simulink library "library_schuettgut"  (R2020a)
settings: Solver=VariableStepAuto  StartTime=0.0  StopTime=10.0  RelTol=1e-3
undefined symbols (not defined in the file or in its folder): delay, gain, OK
libraries: simulink x7, $bdroot x3
settings Model: Creator=Jonathan  LastModifiedBy=Jonathan

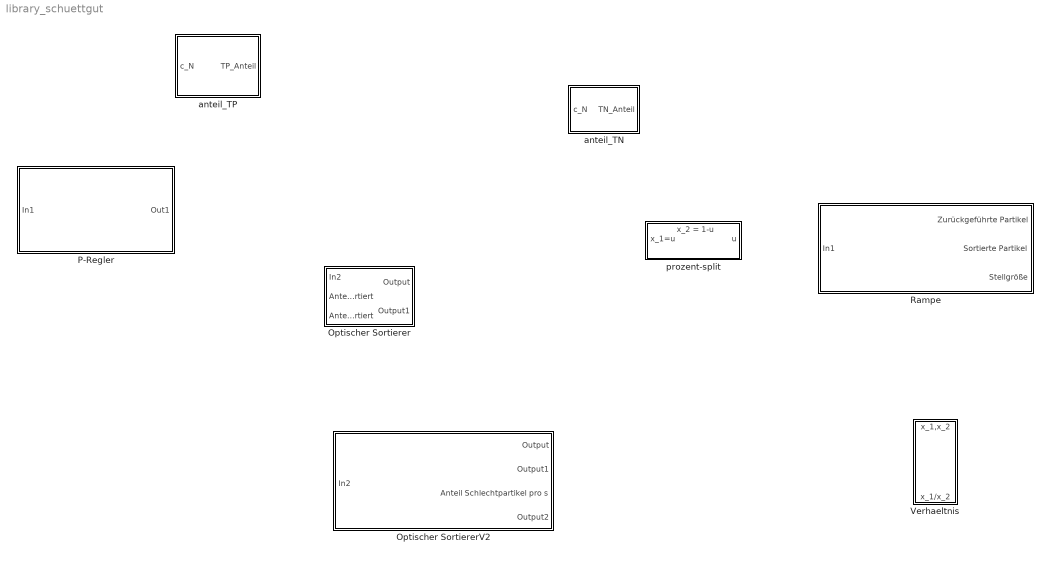
== system library_schuettgut ==
  Optischer Sortierer : Subsystem
  Optischer SortiererV2 : Subsystem  AncestorBlock=library_schuettgut/Optischer Sortierer
  P-Regler : Subsystem  mask{gain=1, delay=1, TrueorFalse=0}
      mask prompts: delay "Time Delay"; TrueorFalse "Reglerinput"
  Rampe : Subsystem  Tag=Rampe  mask{OK=OK, gain=gain, delay=delay, TrueorFalse=0, errorP=0, errorN=0}
      mask prompts: OK "Abstand OS Kamera"; gain "Regler-Gain:"; delay "Regler-Totzeit"; TrueorFalse "Reglerinput:"; errorP "Reglerfehler Gutpartikel:"; errorN "Reglerfehler Schlechtpartikel"
      mask help:
      | Reglerinput:
      | Reglerinput = 1 => Gutpartikel pro s wird als Reglerinput verwendet
      | Reglerinput = 0 => Schlechtpartike pro s wird als Reglerinput verwendet
      mask TypeOptions TrueorFalse: 0 | 1
  "Verhaeltnis " : Subsystem
  anteil_TN : MATLAB Function  TreatAsAtomicUnit=on
  anteil_TP : MATLAB Function  TreatAsAtomicUnit=on
  prozent-split : Subsystem
      settings: PortSchema="{\"entries\":[{\"content\":{\"sides\":[{\"content\":{\"connectorIds\":[\"In1\"]},\"type\":\"ConnectorPlacement.EquallySpacedRectSide\",\"uuid\":\"ab8511c8-9f1d-48ad-bf24-85fd477f0bdd\"},{\"content\":{\"connectorIds\":[\"Out1\"],\"side\":\"RIGHT\"},\"type\":\"ConnectorPlacement.EquallySpacedRectSide\",\"uuid\":\"9ac1a19a-8176-444e-9f4d-7beffa0184e3\"},{\"content\":{\"connectorIds\":[\"Out2\"],\"side\":\"TOP\"},\"type\":\"ConnectorPlacement.EquallySpacedRectSide\",\"uuid\":\"376c2400-f821-4649-ab16-706a2da6117b\"}]},\"type\":\"ConnectorPlacement.EquallySpacedConnector\",\"uuid\":\"f6e72b2d-0467-4732-a018-d51f3a5db703\"}],\"packageUris\":[\"http://schema.mathworks.com/mf0/Connector/19700101\"],\"version\":\"1.0\"}"

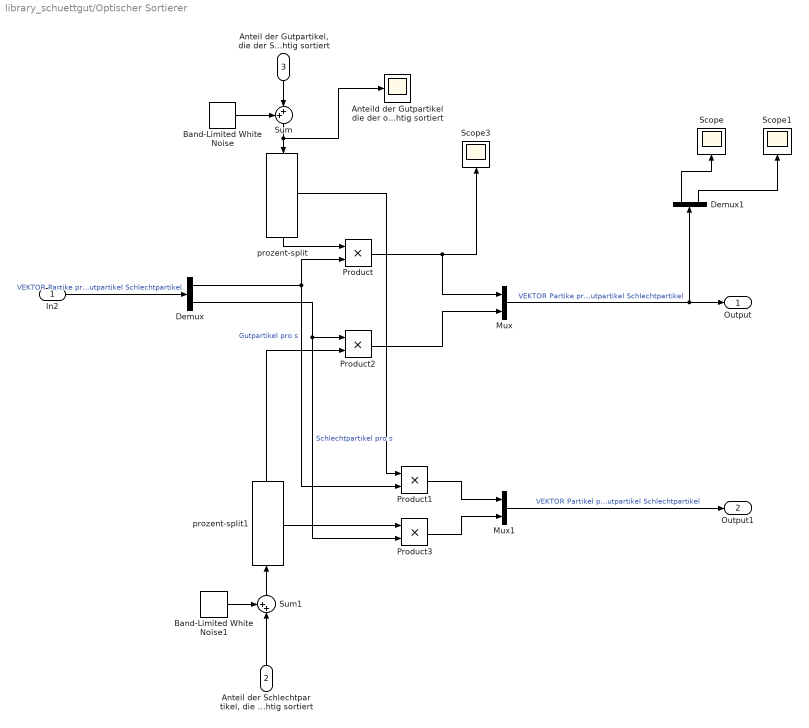
== system library_schuettgut/Optischer Sortierer ==
  In2 : Inport
  "Anteil der Schlechtpartikel, die der Sortierer richtig sortiert " : Inport  Port=2
  "Anteil der Gutpartikel, die der Sortierer richtig sortiert" : Inport  Port=3
  Anteild der Gutpartikel die der optische Sortiererrichtig richtig sortiert : Scope
  Band-Limited White Noise : simulink/Sources/Band-Limited White Noise  Cov=[0.0001]  Ts=0.1  seed=[23341]
  Band-Limited White Noise1 : simulink/Sources/Band-Limited White Noise  Cov=[0.0001]  Ts=0.1  seed=[23341]
  Demux : Demux  Outputs=2
  Demux1 : Demux  Outputs=2
  Mux : Mux  Inputs=2
  Mux1 : Mux  Inputs=2
  Product{,1..3} (4 alike) : Product
  Scope : Scope
  Scope1 : Scope
  Scope3 : Scope
  Sum : Sum  Inputs=++|
  Sum1 : Sum  Inputs=++|
  prozent-split : $bdroot/prozent-split  SystemSampleTime=-1  Latency=0  AutoFrameSizeCalculation=off
      settings: PortSchema="{\"entries\":[{\"content\":{\"sides\":[{\"content\":{\"connectorIds\":[\"In1\"]},\"type\":\"ConnectorPlacement.EquallySpacedRectSide\",\"uuid\":\"ab8511c8-9f1d-48ad-bf24-85fd477f0bdd\"},{\"content\":{\"connectorIds\":[\"Out1\"],\"side\":\"RIGHT\"},\"type\":\"ConnectorPlacement.EquallySpacedRectSide\",\"uuid\":\"9ac1a19a-8176-444e-9f4d-7beffa0184e3\"},{\"content\":{\"connectorIds\":[\"Out2\"],\"side\":\"TOP\"},\"type\":\"ConnectorPlacement.EquallySpacedRectSide\",\"uuid\":\"376c2400-f821-4649-ab16-706a2da6117b\"}]},\"type\":\"ConnectorPlacement.EquallySpacedConnector\",\"uuid\":\"f6e72b2d-0467-4732-a018-d51f3a5db703\"}],\"packageUris\":[\"http://schema.mathworks.com/mf0/Connector/19700101\"],\"version\":\"1.0\"}"
  prozent-split1 : $bdroot/prozent-split  SystemSampleTime=-1  Latency=0  AutoFrameSizeCalculation=off
      settings: PortSchema="{\"entries\":[{\"content\":{\"sides\":[{\"content\":{\"connectorIds\":[\"In1\"]},\"type\":\"ConnectorPlacement.EquallySpacedRectSide\",\"uuid\":\"ab8511c8-9f1d-48ad-bf24-85fd477f0bdd\"},{\"content\":{\"connectorIds\":[\"Out1\"],\"side\":\"RIGHT\"},\"type\":\"ConnectorPlacement.EquallySpacedRectSide\",\"uuid\":\"9ac1a19a-8176-444e-9f4d-7beffa0184e3\"},{\"content\":{\"connectorIds\":[\"Out2\"],\"side\":\"TOP\"},\"type\":\"ConnectorPlacement.EquallySpacedRectSide\",\"uuid\":\"376c2400-f821-4649-ab16-706a2da6117b\"}]},\"type\":\"ConnectorPlacement.EquallySpacedConnector\",\"uuid\":\"f6e72b2d-0467-4732-a018-d51f3a5db703\"}],\"packageUris\":[\"http://schema.mathworks.com/mf0/Connector/19700101\"],\"version\":\"1.0\"}"
  Output : Outport
  Output1 : Outport  Port=2
  wires:
  Demux1/1 -> Scope/1
  Demux1/2 -> Scope1/1
  Product3/1 -> Mux1/2
  Product1/1 -> Mux1/1
  prozent-split1/2 -> Product3/1
  prozent-split1/1 -> Product2/2
  Demux/2 -> Product2/1, Product3/2  "Schlechtpartikel pro s"
  Product2/1 -> Mux/2
  Band-Limited White Noise1/1 -> Sum1/1
  Sum1/1 -> prozent-split1/1
  "Anteil der Schlechtpartikel, die der Sortierer richtig sortiert "/1 -> Sum1/2
  Product/1 -> Mux/1, Scope3/1
  prozent-split/2 -> Product1/1
  Sum/1 -> Anteild der Gutpartikel die der optische Sortiererrichtig richtig sortiert/1, prozent-split/1
  Band-Limited White Noise/1 -> Sum/1
  prozent-split/1 -> Product/1
  Demux/1 -> Product/2, Product1/2  "Gutpartikel pro s"
  Mux/1 -> Output/1, Demux1/1  "VEKTOR Partike pro s in der Gutfraktion: Gutpartikel Schlechtpartikel"
  Mux1/1 -> Output1/1  "VEKTOR Partikel pro s in der Schlechtfraktion: Gutpartikel Schlechtpartikel"
  In2/1 -> Demux/1  "VEKTOR Partike pro s: Gutpartikel Schlechtpartikel"
  "Anteil der Gutpartikel, die der Sortierer richtig sortiert"/1 -> Sum/2

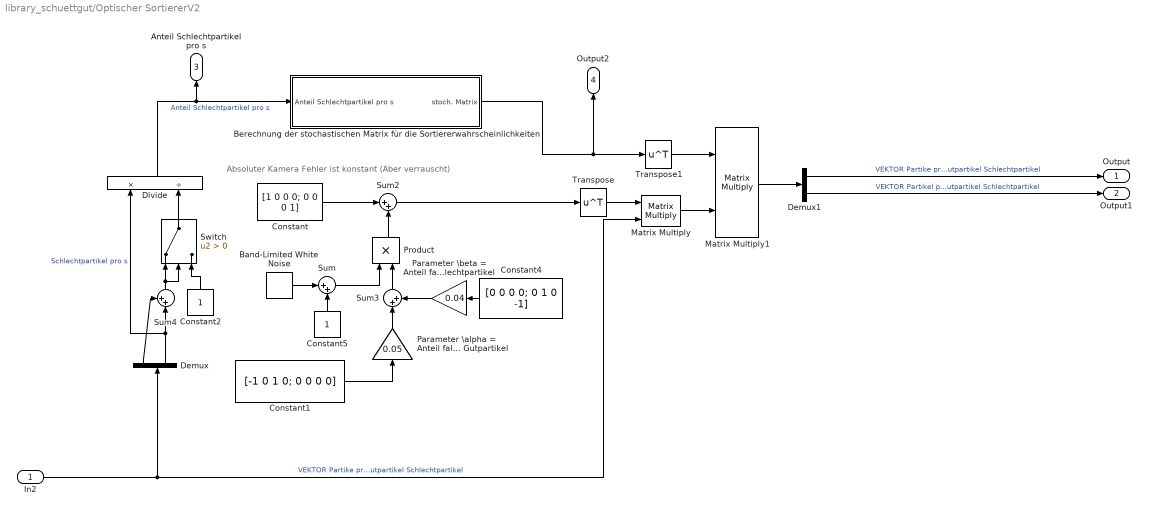
== system library_schuettgut/Optischer SortiererV2 ==
  note: Absoluter Kamera Fehler ist konstant (Aber verrauscht)
  In2 : Inport
  Band-Limited White Noise : simulink/Sources/Band-Limited White Noise  Cov=[0]  Ts=0.1  seed=[23341]
  Berechnung der stochastischen Matrix für die Sortiererwahrscheinlichkeiten : Subsystem
  Constant : Constant  Value=[1 0 0 0; 0 0 0 1]
  Constant1 : Constant  Value=[-1 0 1 0; 0 0 0 0]
  Constant2 : Constant
  Constant4 : Constant  Value=[0 0 0 0; 0 1 0 -1]
  Constant5 : Constant
  Demux : Demux  Outputs=2
  Demux1 : Demux  Outputs=2
  Divide : Product  Inputs=*/
  Matrix Multiply : Product  Multiplication=Matrix(*)
  Matrix Multiply1 : Product  Multiplication=Matrix(*)
  Parameter \alpha = Anteil falsch detektierter Gutpartikel : Gain  Gain=0.05
  Parameter \beta = Anteil falsch detektierter Schlechtpartikel : Gain  Gain=0.04
  Product : Product
  Sum : Sum  Inputs=|++
  Sum2 : Sum  Inputs=|++
  Sum3 : Sum  Inputs=|++
  Sum4 : Sum  Inputs=++|
  Switch : Switch  Criteria=u2 > Threshold
  Transpose : Math  Operator=transpose  SaturateOnIntegerOverflow=on
  Transpose1 : Math  Operator=transpose  SaturateOnIntegerOverflow=on
  Output : Outport
  Output1 : Outport  Port=2
  Anteil Schlechtpartikel pro s : Outport  Port=3
  Output2 : Outport  Port=4
  wires:
  Demux1/1 -> Output/1  "VEKTOR Partike pro s in der Gutfraktion: Gutpartikel Schlechtpartikel"
  Demux1/2 -> Output1/1  "VEKTOR Partikel pro s in der Schlechtfraktion: Gutpartikel Schlechtpartikel"
  Transpose/1 -> Matrix Multiply/1
  Matrix Multiply/1 -> Matrix Multiply1/2
  Transpose1/1 -> Matrix Multiply1/1
  Matrix Multiply1/1 -> Demux1/1
  In2/1 -> Matrix Multiply/2, Demux/1  "VEKTOR Partike pro s: Gutpartikel Schlechtpartikel"
  Constant1/1 -> Parameter \alpha = Anteil falsch detektierter Gutpartikel/1
  Sum2/1 -> Transpose/1
  Demux/2 -> Divide/1, Sum4/2  "Schlechtpartikel pro s"
  Sum4/1 -> Switch/2, Switch/1
  Demux/1 -> Sum4/1
  Divide/1 -> Anteil Schlechtpartikel pro s/1, Berechnung der stochastischen Matrix für die Sortiererwahrscheinlichkeiten/1(Anteil Schlechtpartikel pro s)  "Anteil Schlechtpartikel pro s"
  Berechnung der stochastischen Matrix für die Sortiererwahrscheinlichkeiten/1(stoch. Matrix) -> Output2/1, Transpose1/1
  Constant4/1 -> Parameter \beta = Anteil falsch detektierter Schlechtpartikel/1
  Parameter \beta = Anteil falsch detektierter Schlechtpartikel/1 -> Sum3/2
  Parameter \alpha = Anteil falsch detektierter Gutpartikel/1 -> Sum3/1
  Sum3/1 -> Product/2
  Constant/1 -> Sum2/1
  Product/1 -> Sum2/2
  Sum/1 -> Product/1
  Band-Limited White Noise/1 -> Sum/1
  Constant5/1 -> Sum/2
  Switch/1 -> Divide/2
  Constant2/1 -> Switch/3

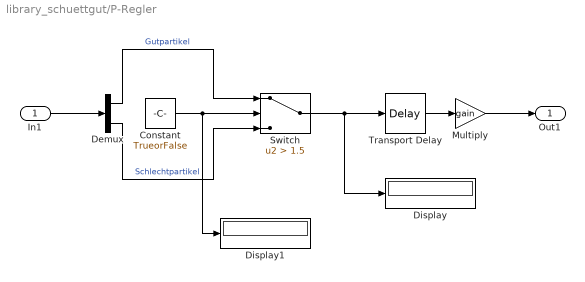
== system library_schuettgut/P-Regler ==
  In1 : Inport
  Constant : Constant  Value=TrueorFalse
  Demux : Demux  Outputs=2
  Display : Display
  Display1 : Display
  Multiply : Gain  Gain=gain
  Switch : Switch  Criteria=u2 > Threshold  Threshold=1.5
  Transport Delay : TransportDelay  DelayTime=delay
  Out1 : Outport
  wires:
  In1/1 -> Demux/1
  Demux/2 -> Switch/3  "Schlechtpartikel"
  Transport Delay/1 -> Multiply/1
  Multiply/1 -> Out1/1
  Constant/1 -> Display1/1, Switch/2
  Demux/1 -> Switch/1  "Gutpartikel"
  Switch/1 -> Display/1, Transport Delay/1

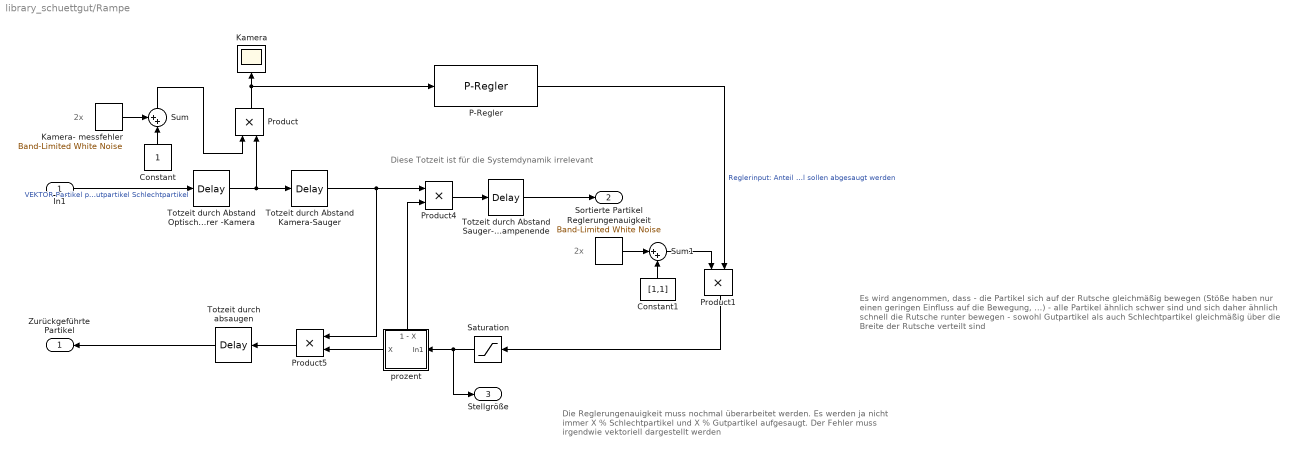
== system library_schuettgut/Rampe ==
  note: Diese Totzeit ist für die Systemdynamik irrelevant
  note: 2x
  note: 2x
  note: Die Reglerungenauigkeit muss nochmal überarbeitet werden.
      | Es werden ja nicht immer X % Schlechtpartikel und X %
      | Gutpartikel aufgesaugt. Der Fehler muss irgendwie vektoriell dargestellt werden
  note: Es wird angenommen, dass
      | - die Partikel sich auf der Rutsche gleichmäßig bewegen (Stöße haben nur einen geringen Einfluss auf die Bewegung, ...)
      | - alle Partikel ähnlich schwer sind und sich daher ähnlich schnell die Rutsche runter bewegen
      | - sowohl Gutpartikel als auch Schlechtpartikel gleichmäßig über die Breite der Rutsche verteilt sind
  In1 : Inport
  Constant : Constant
  Constant1 : Constant  Value=[1,1]
  Kamera : Scope
  Kamera- messfehler : simulink/Sources/Band-Limited White Noise  Cov=[0.0001 0.00011]  Ts=0.1  seed=[23341]
  P-Regler : $bdroot/P-Regler  gain=gain  delay=delay  TrueorFalse=TrueorFalse
  Product : Product
  Product1 : Product  OutMin=0  OutMax=1
  Product4 : Product
  Product5 : Product
  Reglerungenauigkeit : simulink/Sources/Band-Limited White Noise  Cov=[errorP errorN]  Ts=0.1  seed=[23341]
  Saturation : Saturate  UpperLimit=0.9  LowerLimit=0
  Sum : Sum  Inputs=++|
  Sum1 : Sum  Inputs=|++
  Totzeit durch Abstand Optischer Sortierer -Kamera : TransportDelay  DelayTime=OK
  Totzeit durch Abstand Kamera-Sauger : TransportDelay
  Totzeit durch Abstand Sauger-Rampenende : TransportDelay
  Totzeit durch absaugen : TransportDelay
  prozent : Subsystem
      settings: PortSchema="{\"entries\":[{\"content\":{\"sides\":[{\"content\":{\"connectorIds\":[\"In1\"]},\"type\":\"ConnectorPlacement.EquallySpacedRectSide\",\"uuid\":\"ab8511c8-9f1d-48ad-bf24-85fd477f0bdd\"},{\"content\":{\"connectorIds\":[\"Out1\"],\"side\":\"RIGHT\"},\"type\":\"ConnectorPlacement.EquallySpacedRectSide\",\"uuid\":\"9ac1a19a-8176-444e-9f4d-7beffa0184e3\"},{\"content\":{\"connectorIds\":[\"Out2\"],\"side\":\"TOP\"},\"type\":\"ConnectorPlacement.EquallySpacedRectSide\",\"uuid\":\"376c2400-f821-4649-ab16-706a2da6117b\"}]},\"type\":\"ConnectorPlacement.EquallySpacedConnector\",\"uuid\":\"f6e72b2d-0467-4732-a018-d51f3a5db703\"}],\"packageUris\":[\"http://schema.mathworks.com/mf0/Connector/19700101\"],\"version\":\"1.0\"}"
  Zurückgeführte Partikel : Outport
  Sortierte Partikel : Outport  Port=2
  Stellgröße : Outport  Port=3
  wires:
  prozent/2(1 - X) -> Product4/2
  prozent/1(X) -> Product5/2
  In1/1 -> Totzeit durch Abstand Optischer Sortierer -Kamera/1  "VEKTOR Partikel pro s: Gutpartikel Schlechtpartikel"
  Product/1 -> Kamera/1, P-Regler/1
  Totzeit durch absaugen/1 -> Zurückgeführte Partikel/1
  Totzeit durch Abstand Optischer Sortierer -Kamera/1 -> Totzeit durch Abstand Kamera-Sauger/1, Product/2
  Product5/1 -> Totzeit durch absaugen/1
  Totzeit durch Abstand Kamera-Sauger/1 -> Product4/1, Product5/1
  Totzeit durch Abstand Sauger-Rampenende/1 -> Sortierte Partikel/1
  Kamera- messfehler/1 -> Sum/1
  Product4/1 -> Totzeit durch Abstand Sauger-Rampenende/1
  P-Regler/1 -> Product1/2  "Reglerinput: Anteil X der Partikel sollen abgesaugt werden"
  Constant/1 -> Sum/2
  Sum/1 -> Product/1
  Reglerungenauigkeit/1 -> Sum1/1
  Constant1/1 -> Sum1/2
  Product1/1 -> Saturation/1
  Saturation/1 -> Stellgröße/1, prozent/1(In1)
  Sum1/1 -> Product1/1

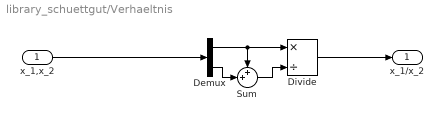
== system library_schuettgut/Verhaeltnis  ==
  x_1,x_2 : Inport
  Demux : Demux  Outputs=2
  Divide : Product  Inputs=*/
  Sum : Sum  Inputs=++|
  x_1/x_2 : Outport
  wires:
  Divide/1 -> x_1/x_2/1
  Demux/2 -> Sum/2
  Demux/1 -> Divide/1, Sum/1
  x_1,x_2/1 -> Demux/1
  Sum/1 -> Divide/2

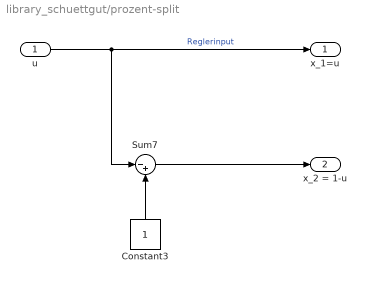
== system library_schuettgut/prozent-split ==
  u : Inport
  Constant3 : Constant
  Sum7 : Sum  Inputs=|-+
  x_1=u : Outport
  x_2 = 1-u : Outport  Port=2
  wires:
  Constant3/1 -> Sum7/2
  u/1 -> Sum7/1, x_1=u/1  "Reglerinput"
  Sum7/1 -> x_2 = 1-u/1

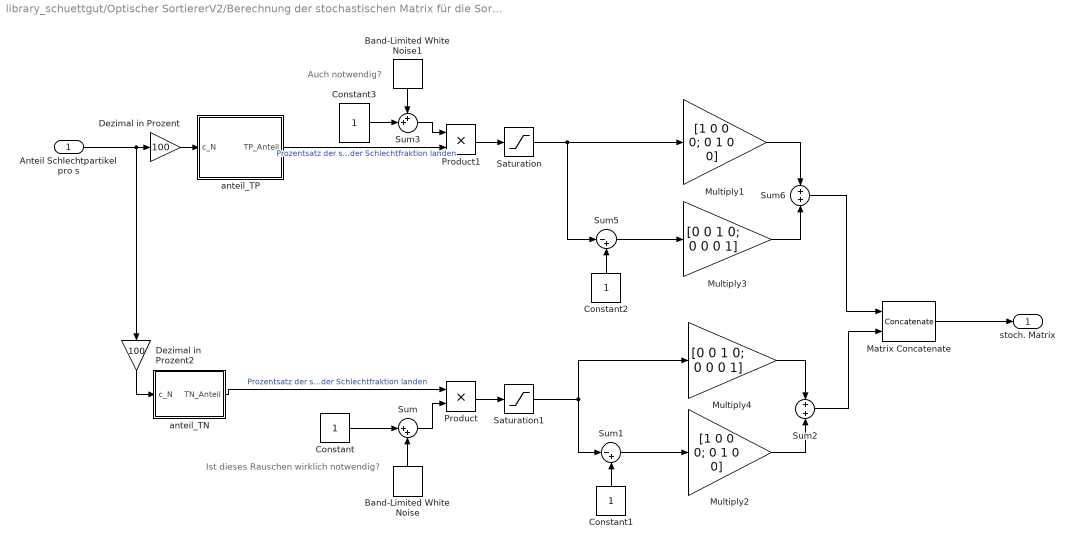
== system library_schuettgut/Optischer SortiererV2/Berechnung der stochastischen Matrix für die Sortiererwahrscheinlichkeiten ==
  note: Auch notwendig?
  note: Ist dieses Rauschen wirklich notwendig?
  Anteil Schlechtpartikel pro s : Inport
  Band-Limited White Noise : simulink/Sources/Band-Limited White Noise  Cov=[0]  Ts=0.1  seed=[23341]
  Band-Limited White Noise1 : simulink/Sources/Band-Limited White Noise  Cov=[0]  Ts=0.1  seed=[23341]
  Constant{,1..3} (4 alike) : Constant
  Dezimal in Prozent : Gain  Gain=100
  Dezimal in Prozent2 : Gain  Gain=100
  Matrix Concatenate : Concatenate  Mode=Multidimensional array
  Multiply1 : Gain  Gain=[1 0 0 0; 0 1 0 0]
  Multiply2 : Gain  Gain=[1 0 0 0; 0 1 0 0]
  Multiply3 : Gain  Gain=[0 0 1 0; 0 0 0 1]
  Multiply4 : Gain  Gain=[0 0 1 0; 0 0 0 1]
  Product : Product
  Product1 : Product
  Saturation : Saturate  UpperLimit=1  LowerLimit=0
  Saturation1 : Saturate  UpperLimit=1  LowerLimit=0
  Sum : Sum  Inputs=|++
  Sum1 : Sum  Inputs=|-+
  Sum2 : Sum  Inputs=+|+
  Sum3 : Sum  Inputs=++|
  Sum5 : Sum  Inputs=|-+
  Sum6 : Sum  Inputs=+|+
  anteil_TN : MATLAB Function  TreatAsAtomicUnit=on
  anteil_TP : MATLAB Function  TreatAsAtomicUnit=on
  stoch. Matrix : Outport
  wires:
  Multiply3/1 -> Sum6/2
  Sum5/1 -> Multiply3/1
  Constant2/1 -> Sum5/2
  Sum1/1 -> Multiply2/1
  Constant1/1 -> Sum1/2
  Multiply2/1 -> Sum2/2
  Multiply4/1 -> Sum2/1
  Anteil Schlechtpartikel pro s/1 -> Dezimal in Prozent/1, Dezimal in Prozent2/1
  Multiply1/1 -> Sum6/1
  Matrix Concatenate/1 -> stoch. Matrix/1
  Sum2/1 -> Matrix Concatenate/2
  Sum6/1 -> Matrix Concatenate/1
  Saturation1/1 -> Multiply4/1, Sum1/1
  Saturation/1 -> Sum5/1, Multiply1/1
  Dezimal in Prozent/1 -> anteil_TP/1(c_N)
  Dezimal in Prozent2/1 -> anteil_TN/1(c_N)
  Sum/1 -> Product/2
  Constant/1 -> Sum/1
  Sum3/1 -> Product1/1
  Constant3/1 -> Sum3/2
  anteil_TN/1(TN_Anteil) -> Product/1  "Prozentsatz der schlecht detektierten Partikel, die in der Schlechtfraktion landen"
  anteil_TP/1(TP_Anteil) -> Product1/2  "Prozentsatz der schlecht detektierten Partikel, die in der Schlechtfraktion landen"
  Band-Limited White Noise1/1 -> Sum3/1
  Product1/1 -> Saturation/1
  Product/1 -> Saturation1/1
  Band-Limited White Noise/1 -> Sum/2

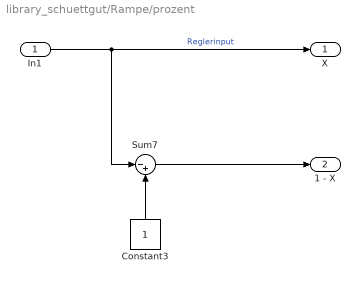
== system library_schuettgut/Rampe/prozent ==
  In1 : Inport
  Constant3 : Constant
  Sum7 : Sum  Inputs=|-+
  X : Outport
  1 - X : Outport  Port=2
  wires:
  Constant3/1 -> Sum7/2
  In1/1 -> Sum7/1, X/1  "Reglerinput"
  Sum7/1 -> 1 - X/1

== matlab function library_schuettgut/anteil_TP ==
  data: c_N input; TP_Anteil output
function TP_Anteil = anteil_TP(c_N)
%#codegen

%    This function was generated by the Symbolic Math Toolbox version 8.5.
%    23-Nov-2020 21:35:04

t2 = c_N.^2;
t3 = c_N.*1.216152772820919e-1;
t5 = c_N.*1.718305977216851e-4;
t4 = exp(t3);
t6 = -t5;
t7 = exp(t6);
t8 = t4.*3.965528248105649e+15;
t9 = t7.*2.950835993543266e+20;
t10 = -t9;
TP_Anteil = ((t8+t10).*(c_N.*2.712794053385412e+19+t2.*1.147738374932383e+17-3.299572958664278e+21).*1.965116437629977e-18)./((c_N.*(1.45e+2./2.0)-7.25e+3).*(c_N.*-7.812438090851985e+17+t2.*9.181906999459062e+15+t8+t10+3.118206848621062e+19));

== matlab function library_schuettgut/anteil_TN ==
  data: c_N input; TN_Anteil output
function TN_Anteil = anteil_TN(c_N)
%#codegen

%    This function was generated by the Symbolic Math Toolbox version 8.5.
%    23-Nov-2020 21:38:40

t2 = c_N.^2;
t3 = c_N.*1.216152772820919e-1;
t5 = c_N.*1.718305977216851e-4;
t4 = exp(t3);
t6 = -t5;
t7 = exp(t6);
TN_Anteil = ((c_N.*3.906219045425992e+17-t2.*4.590953499729531e+15+1.319829183465711e+20).*(c_N.*7.378697629483821e+19-t4.*9.913820620264122e+16+t7.*7.377089983858165e+21-7.378697629483821e+21).*(-2.710505431213761e-20))./(c_N.*(c_N.*-7.812438090851985e+17+t2.*9.181906999459062e+15+t4.*3.965528248105649e+15-t7.*2.950835993543266e+20+3.118206848621062e+19));

== matlab function library_schuettgut/Optischer SortiererV2/Berechnung der stochastischen Matrix für die Sortiererwahrscheinlichkeiten/anteil_TN ==
  data: c_N input; TN_Anteil output
function TN_Anteil = anteil_TN(c_N)
%#codegen

%    This function was generated by the Symbolic Math Toolbox version 8.5.
%    23-Nov-2020 21:38:40

t2 = c_N.^2;
t3 = c_N.*1.216152772820919e-1;
t5 = c_N.*1.718305977216851e-4;
t4 = exp(t3);
t6 = -t5;
t7 = exp(t6);
TN_Anteil = ((c_N.*3.906219045425992e+17-t2.*4.590953499729531e+15+1.319829183465711e+20).*(c_N.*7.378697629483821e+19-t4.*9.913820620264122e+16+t7.*7.377089983858165e+21-7.378697629483821e+21).*(-2.710505431213761e-20))./(c_N.*(c_N.*-7.812438090851985e+17+t2.*9.181906999459062e+15+t4.*3.965528248105649e+15-t7.*2.950835993543266e+20+3.118206848621062e+19));

== matlab function library_schuettgut/Optischer SortiererV2/Berechnung der stochastischen Matrix für die Sortiererwahrscheinlichkeiten/anteil_TP ==
  data: c_N input; TP_Anteil output
function TP_Anteil = anteil_TP(c_N)
%#codegen

%    This function was generated by the Symbolic Math Toolbox version 8.5.
%    23-Nov-2020 21:35:04

t2 = c_N.^2;
t3 = c_N.*1.216152772820919e-1;
t5 = c_N.*1.718305977216851e-4;
t4 = exp(t3);
t6 = -t5;
t7 = exp(t6);
t8 = t4.*3.965528248105649e+15;
t9 = t7.*2.950835993543266e+20;
t10 = -t9;
TP_Anteil = ((t8+t10).*(c_N.*2.712794053385412e+19+t2.*1.147738374932383e+17-3.299572958664278e+21).*1.965116437629977e-18)./((c_N.*(1.45e+2./2.0)-7.25e+3).*(c_N.*-7.812438090851985e+17+t2.*9.181906999459062e+15+t8+t10+3.118206848621062e+19));
